simulink model "Turntable_sweep_close"  (R2017b)
settings: Solver=FixedStepAuto  StartTime=0.0  StopTime=10.0  FixedStep=0.0005  RelTol=1e-3
values from neighbouring files (symbols this model uses):
  fre = fre_array(i)    [sweep.m]    (also in sweep_close.m; turntable_friction.mat = 150)
  mag = 1    [sweep.m]    (also in sweep_close.m; test.m = ET205(1: 75, 1); turntable_friction.mat = 5)
  t_off = 10    [sweep.m]    (also in sweep_close.m; turntable_friction.mat)
settings Model: Creator=Vera  LastModifiedBy=surunbing
settings OptimizationCC: LifeSpan=inf
settings DebuggingCC: SFExecutionAtInitializationDiag=none
settings CodeAppCC: StateflowObjectComments=on

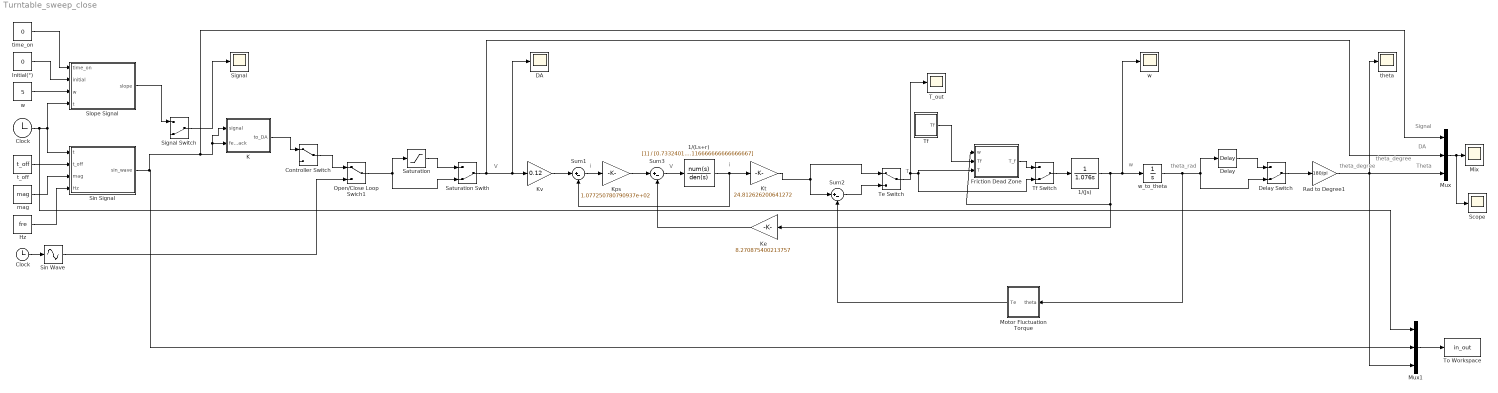
== system Turntable_sweep_close ==
  note: w
  note: theta_degree
  note: theta_rad
  note: T
  note: V
  note: i
  note: i
  note: V
  note: Signal
  note: DA
  note: Theta
  note: theta_degree
  " Delay Switch" : ManualSwitch  CurrentSetting=0
  1/(Js) : TransferFcn  Denominator=[1.076 0]
  1/(Ls+r) : TransferFcn  Denominator=[0.733240176511722 80.116666666666666667]
  Clock : Clock
  "Clock   " : Clock
  Controller Switch : ManualSwitch
  DA : Scope
  Delay : TransportDelay  DelayTime=0.003763900000000
  Friction Dead Zone : MATLAB Function  TreatAsAtomicUnit=on
  Hz : Constant  Value=fre
  Initial(°) : Constant  Value=0
  K : Subsystem
  Ke : Gain  Gain=8.270875400213757
  Kps : Gain  Gain=1.077250780790937e+02
  Kt : Gain  Gain=24.812626200641272
  Kv : Gain  Gain=0.12
  Mix : Scope
  Motor Fluctuation Torque : Subsystem
  Mux : Mux  Inputs=3
  Mux1 : Mux  Inputs=3
  Open/Close Loop Swich1 : ManualSwitch
  Rad to Degree1 : Gain  Gain=180/pi
  Saturation : Saturate  UpperLimit=10  LowerLimit=-10
  Saturation Swith : ManualSwitch  CurrentSetting=0
  Scope : Scope
  Signal : Scope
  Signal Switch : ManualSwitch  CurrentSetting=0
  Sin Signal : MATLAB Function  TreatAsAtomicUnit=on
  Sin Wave : Sin  TimeSource=Use external signal  Amplitude=0  Bias=5  Frequency=0.05*2*pi  SampleTime=0
  Slope Signal : MATLAB Function  TreatAsAtomicUnit=on
  Sum1 : Sum  Inputs=|+-
  Sum2 : Sum  Inputs=|+-
  Sum3 : Sum  Inputs=|+-
  T_out : Scope
  Te Switch : ManualSwitch
  Tf : Subsystem
  Tf Switch : ManualSwitch  CurrentSetting=0
  To Workspace : ToWorkspace  VariableName=in_out  SampleTime=-1
  mag : Constant  Value=mag
  t_off : Constant  Value=t_off
  theta : Scope
  time_on : Constant  Value=0
  w : Constant  Value=5
  "w " : Scope
  w_to_theta : Integrator
  wires:
  Sum1/1 -> Kps/1
  Delay/1 -> " Delay Switch"/1
  Ke/1 -> Sum3/2
  Te Switch/1 -> T_out/1, Tf Switch/2, Friction Dead Zone/3(T)
  Kps/1 -> Sum3/1
  Kt/1 -> Te Switch/1, Sum2/1
  Sum3/1 -> 1/(Ls+r)/1
  1/(Ls+r)/1 -> Kt/1, Sum1/2
  Kv/1 -> Sum1/1
  1/(Js)/1 -> Ke/1, Friction Dead Zone/1(w), w_to_theta/1, "w "/1
  Motor Fluctuation Torque/1(Te) -> Sum2/2
  w_to_theta/1 -> Delay/1, " Delay Switch"/2, Motor Fluctuation Torque/1(theta)
  Sum2/1 -> Te Switch/2
  Friction Dead Zone/1(T_f) -> Tf Switch/1
  Tf Switch/1 -> 1/(Js)/1
  Sin Signal/1(sin_wave) -> Mux/1, K/1(signal), K/2(feedback), Mux1/2
  Signal Switch/1 -> Signal/1
  K/1(to_DA) -> Controller Switch/1
  t_off/1 -> Sin Signal/2(t_off)
  Clock/1 -> Mux1/1, Sin Signal/1(t), Slope Signal/4(t)
  mag/1 -> Sin Signal/3(mag)
  Hz/1 -> Sin Signal/4(Hz)
  Controller Switch/1 -> Open/Close Loop Swich1/1
  Sin Wave/1 -> Open/Close Loop Swich1/2
  time_on/1 -> Slope Signal/1(time_on)
  Initial(°)/1 -> Slope Signal/2(initial)
  w/1 -> Slope Signal/3(w)
  Slope Signal/1(slope) -> Signal Switch/1
  "Clock   "/1 -> Sin Wave/1
  Rad to Degree1/1 -> Mux1/3, theta/1, Mux/3
  Saturation/1 -> Saturation Swith/1
  Open/Close Loop Swich1/1 -> Saturation/1, Saturation Swith/2
  Saturation Swith/1 -> Mux/2, DA/1, Kv/1
  Mux/1 -> Scope/1, Mix/1
  " Delay Switch"/1 -> Rad to Degree1/1
  Tf/1(Tf) -> Friction Dead Zone/2(Tf)
  Mux1/1 -> To Workspace/1

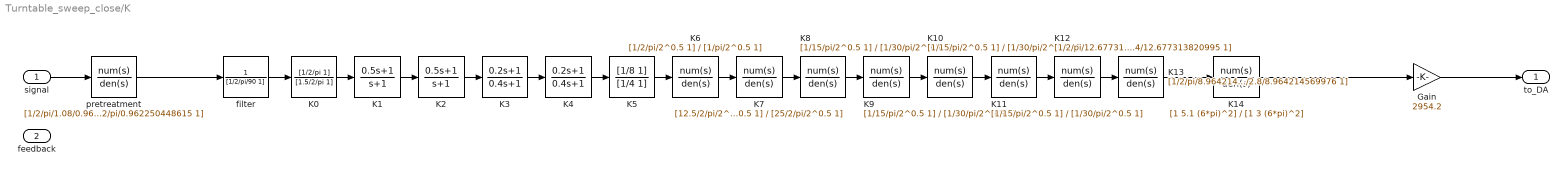
== system Turntable_sweep_close/K ==
  signal : Inport
  feedback : Inport  Port=2
  Gain : Gain  Gain=2954.2
  K0 : TransferFcn  Numerator=[1/2/pi 1]  Denominator=[1.5/2/pi 1]
  K1 : TransferFcn  Numerator=[0.5 1]  Denominator=[1 1]
  K{8..11} (4 alike) : TransferFcn  Numerator=[1/15/pi/2^0.5 1]  Denominator=[1/30/pi/2^0.5 1]
  K12 : TransferFcn  Numerator=[1/2/pi/12.677313820995 1]  Denominator=[1/2/pi/1.4/12.677313820995 1]
  K13 : TransferFcn  Numerator=[1/2/pi/8.964214569976 1]  Denominator=[1/2/pi/2.8/8.964214569976 1]
  K14 : TransferFcn  Numerator=[1 5.1 (6*pi)^2]  Denominator=[1 3 (6*pi)^2]
  K2 : TransferFcn  Numerator=[0.5 1]  Denominator=[1 1]
  K3 : TransferFcn  Numerator=[0.2 1]  Denominator=[0.4 1]
  K4 : TransferFcn  Numerator=[0.2 1]  Denominator=[0.4 1]
  K5 : TransferFcn  Numerator=[1/8 1]  Denominator=[1/4 1]
  K6 : TransferFcn  Numerator=[1/2/pi/2^0.5 1]  Denominator=[1/pi/2^0.5 1]
  K7 : TransferFcn  Numerator=[12.5/2/pi/2^0.5 1]  Denominator=[25/2/pi/2^0.5 1]
  filter : TransferFcn  Numerator=[0 1]  Denominator=[1/2/pi/90 1]
  pretreatment : TransferFcn  Numerator=[1/2/pi/1.08/0.962250448615 1]  Denominator=[1/2/pi/0.962250448615 1]
  to_DA : Outport
  wires:
  K13/1 -> K14/1
  K12/1 -> K13/1
  K11/1 -> K12/1
  K10/1 -> K11/1
  K9/1 -> K10/1
  K8/1 -> K9/1
  K7/1 -> K8/1
  K6/1 -> K7/1
  K5/1 -> K6/1
  K4/1 -> K5/1
  K3/1 -> K4/1
  K2/1 -> K3/1
  K1/1 -> K2/1
  K0/1 -> K1/1
  signal/1 -> pretreatment/1
  pretreatment/1 -> filter/1
  filter/1 -> K0/1
  K14/1 -> Gain/1
  Gain/1 -> to_DA/1

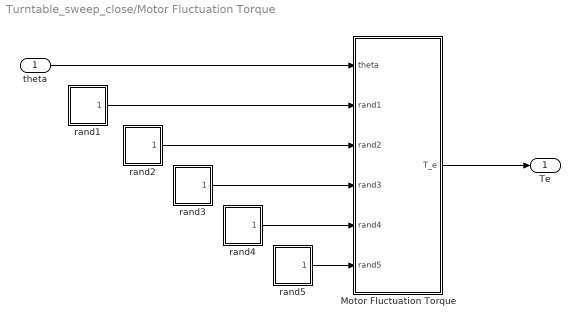
== system Turntable_sweep_close/Motor Fluctuation Torque ==
  theta : Inport
  Motor Fluctuation Torque : MATLAB Function  TreatAsAtomicUnit=on
  rand1 : Subsystem
  rand2 : Subsystem
  rand3 : Subsystem
  rand4 : Subsystem
  rand5 : Subsystem
  Te : Outport
  wires:
  theta/1 -> Motor Fluctuation Torque/1(theta)
  rand1/1(rand1) -> Motor Fluctuation Torque/2(rand1)
  rand2/1(rand2) -> Motor Fluctuation Torque/3(rand2)
  rand3/1(rand3) -> Motor Fluctuation Torque/4(rand3)
  rand4/1(rand4) -> Motor Fluctuation Torque/5(rand4)
  rand5/1(rand5) -> Motor Fluctuation Torque/6(rand5)
  Motor Fluctuation Torque/1(T_e) -> Te/1

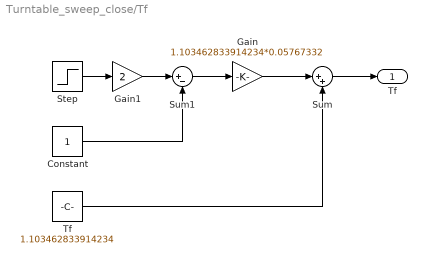
== system Turntable_sweep_close/Tf ==
  Constant : Constant
  Gain : Gain  Gain=1.103462833914234*0.05767332
  Gain1 : Gain  Gain=2
  Step : Step  Time=0  After=rand  SampleTime=0
  Sum : Sum  Inputs=|++
  Sum1 : Sum  Inputs=|+-
  "Tf " : Constant  Value=1.103462833914234
  Tf : Outport
  wires:
  Gain/1 -> Sum/1
  "Tf "/1 -> Sum/2
  Sum/1 -> Tf/1
  Step/1 -> Gain1/1
  Gain1/1 -> Sum1/1
  Constant/1 -> Sum1/2
  Sum1/1 -> Gain/1

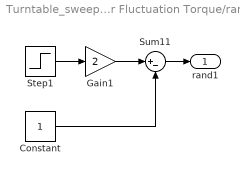
== system Turntable_sweep_close/Motor Fluctuation Torque/rand1 ==
  Constant : Constant
  Gain1 : Gain  Gain=2
  Step1 : Step  Time=0  After=rand  SampleTime=0
  Sum11 : Sum  Inputs=|+-
  rand1 : Outport
  wires:
  Step1/1 -> Gain1/1
  Gain1/1 -> Sum11/1
  Constant/1 -> Sum11/2
  Sum11/1 -> rand1/1

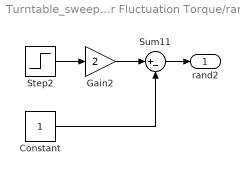
== system Turntable_sweep_close/Motor Fluctuation Torque/rand2 ==
  Constant : Constant
  Gain2 : Gain  Gain=2
  Step2 : Step  Time=0  After=rand  SampleTime=0
  Sum11 : Sum  Inputs=|+-
  rand2 : Outport
  wires:
  Step2/1 -> Gain2/1
  Gain2/1 -> Sum11/1
  Constant/1 -> Sum11/2
  Sum11/1 -> rand2/1

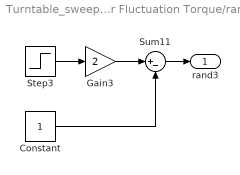
== system Turntable_sweep_close/Motor Fluctuation Torque/rand3 ==
  Constant : Constant
  Gain3 : Gain  Gain=2
  Step3 : Step  Time=0  After=rand  SampleTime=0
  Sum11 : Sum  Inputs=|+-
  rand3 : Outport
  wires:
  Sum11/1 -> rand3/1
  Constant/1 -> Sum11/2
  Gain3/1 -> Sum11/1
  Step3/1 -> Gain3/1

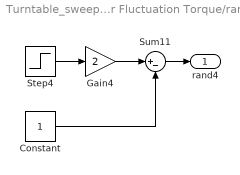
== system Turntable_sweep_close/Motor Fluctuation Torque/rand4 ==
  Constant : Constant
  Gain4 : Gain  Gain=2
  Step4 : Step  Time=0  After=rand  SampleTime=0
  Sum11 : Sum  Inputs=|+-
  rand4 : Outport
  wires:
  Step4/1 -> Gain4/1
  Gain4/1 -> Sum11/1
  Constant/1 -> Sum11/2
  Sum11/1 -> rand4/1

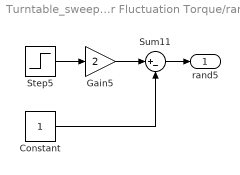
== system Turntable_sweep_close/Motor Fluctuation Torque/rand5 ==
  Constant : Constant
  Gain5 : Gain  Gain=2
  Step5 : Step  Time=0  After=rand  SampleTime=0
  Sum11 : Sum  Inputs=|+-
  rand5 : Outport
  wires:
  Sum11/1 -> rand5/1
  Constant/1 -> Sum11/2
  Gain5/1 -> Sum11/1
  Step5/1 -> Gain5/1

== matlab function Turntable_sweep_close/Sin Signal ==
  data: t input; t_off input; mag input; sin_wave output; Hz input
function sin_wave = fcn(t,t_off,mag,Hz)
w=2*pi*Hz;
if((t>=0)&&(t<1))
    sin_wave=t*mag*sin(w*t);
elseif((t>=1)&&(t<t_off-1))
    sin_wave=mag*sin(w*t);
elseif((t>=(t_off-1))&&(t<t_off))
    sin_wave=-mag*(t-t_off)*sin(w*t);
else
    sin_wave=0;
end

== matlab function Turntable_sweep_close/Friction Dead Zone ==
  data: w input; Tf input; T input; T_f output
function T_f = fcn(w,Tf,T)
if w==0
    if abs(T)<abs(Tf)
        T_f = 0;
    else
        T_f=sign(T)*(abs(T)-Tf);
    end
elseif w*T<0
    T_f=sign(T)*(abs(T)+Tf);
else 
        if abs(T)<abs(Tf)
            T_f = -sign(w)*(Tf-abs(T));
        else
            T_f=sign(T)*(abs(T)-Tf);
        end

end
end

== matlab function Turntable_sweep_close/Slope Signal ==
  data: time_on input; initial input; w input; t input; slope output
function slope = fcn(time_on,initial,w,t)
if t<time_on
    slope=initial;
else
    slope=initial+(t-time_on)*w;
end
end

== matlab function Turntable_sweep_close/Motor Fluctuation Torque/Motor Fluctuation Torque ==
  data: T_e output; theta input; rand1 input; rand2 input; rand3 input; rand4 input; rand5 input
function T_e = fcn(theta,rand1,rand2,rand3,rand4,rand5)
T_p =0.432273269433135*(1+rand1*0.012015015613962)*cos(theta*7 +(48.13841636+0.050850865438431)*pi/180);
T_2p=0.035501355062786*(1+rand2*0.032198449030114)*cos(theta*14+(30.38979755+0.101746126073106)*pi/180);
T_4p=0.018930935537422*(1+rand3*0.028225982587057)*cos(theta*28+(285.7823597+0.203848223609672)*pi/180);
T_6p=0.012218243879728*(1+rand4*0.058230694793342)*cos(theta*42+(152.9148096+0.306666606518932)*pi/180);
T_45=0.009203318745614*(1+rand5*0.098213466988815)*cos(theta*45+(279.6898495+0.328827530537396)*pi/180);

T_e=T_p + T_2p + T_4p + T_6p + T_45;
end
